simulink model "Par10_3_3S"  (R2018a)
settings: Solver=ode3  StartTime=0.0  StopTime=10.0  FixedStep=0.001  RelTol=1e-3
settings Model: Creator=wangluo  LastModifiedBy=wangluo

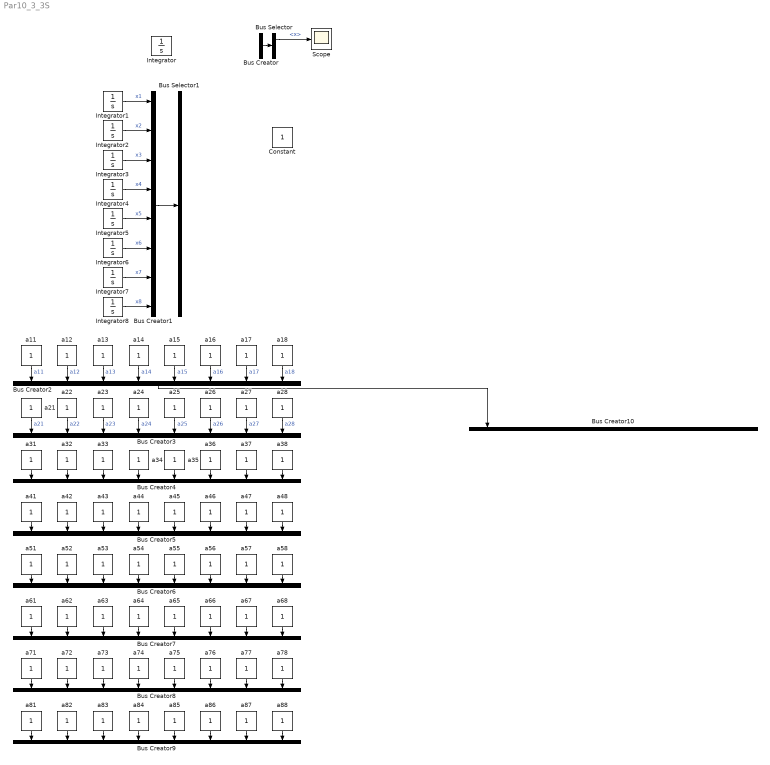
== system Par10_3_3S ==
  Bus Creator : BusCreator  Inputs=2
  Bus Creator{1..10} (10 alike) : BusCreator  Inputs=8
  Bus Selector : BusSelector  OutputSignals=x,signal2
  Bus Selector1 : BusSelector  OutputSignals=x1,x2,x3,x4,x5,x6,x7,x8
  Constant : Constant
  Integrator : Integrator  InitialCondition=[10, 4, 8, 2, 9, 3, 5, 7]
  Integrator{1..8} (8 alike) : Integrator  InitialCondition=[1, 2]
  Scope : Scope
  a{11..18,21..28,31..38,41..48,51..58,61..68,71..78,81..88} (64 alike) : Constant
  wires:
  Bus Selector/1 -> Scope/1  "<x>"
  Bus Creator/1 -> Bus Selector/1
  Integrator1/1 -> Bus Creator1/1  "x1"
  Integrator8/1 -> Bus Creator1/8  "x8"
  Integrator7/1 -> Bus Creator1/7  "x7"
  Integrator6/1 -> Bus Creator1/6  "x6"
  Integrator5/1 -> Bus Creator1/5  "x5"
  Integrator4/1 -> Bus Creator1/4  "x4"
  Integrator3/1 -> Bus Creator1/3  "x3"
  Integrator2/1 -> Bus Creator1/2  "x2"
  Bus Creator1/1 -> Bus Selector1/1
  a11/1 -> Bus Creator2/1  "a11"
  a12/1 -> Bus Creator2/2  "a12"
  a13/1 -> Bus Creator2/3  "a13"
  a14/1 -> Bus Creator2/4  "a14"
  a15/1 -> Bus Creator2/5  "a15"
  a16/1 -> Bus Creator2/6  "a16"
  a17/1 -> Bus Creator2/7  "a17"
  a18/1 -> Bus Creator2/8  "a18"
  a22/1 -> Bus Creator3/2  "a22"
  a24/1 -> Bus Creator3/4  "a24"
  a26/1 -> Bus Creator3/6  "a26"
  a28/1 -> Bus Creator3/8  "a28"
  a25/1 -> Bus Creator3/5  "a25"
  a27/1 -> Bus Creator3/7  "a27"
  a23/1 -> Bus Creator3/3  "a23"
  a21/1 -> Bus Creator3/1  "a21"
  a38/1 -> Bus Creator4/8
  a33/1 -> Bus Creator4/3
  a34/1 -> Bus Creator4/4
  a35/1 -> Bus Creator4/5
  a32/1 -> Bus Creator4/2
  a36/1 -> Bus Creator4/6
  a37/1 -> Bus Creator4/7
  a31/1 -> Bus Creator4/1
  a42/1 -> Bus Creator5/2
  a44/1 -> Bus Creator5/4
  a46/1 -> Bus Creator5/6
  a48/1 -> Bus Creator5/8
  a45/1 -> Bus Creator5/5
  a47/1 -> Bus Creator5/7
  a43/1 -> Bus Creator5/3
  a41/1 -> Bus Creator5/1
  a52/1 -> Bus Creator6/2
  a55/1 -> Bus Creator6/5
  a56/1 -> Bus Creator6/6
  a53/1 -> Bus Creator6/3
  a54/1 -> Bus Creator6/4
  a57/1 -> Bus Creator6/7
  a58/1 -> Bus Creator6/8
  a51/1 -> Bus Creator6/1
  a62/1 -> Bus Creator7/2
  a65/1 -> Bus Creator7/5
  a63/1 -> Bus Creator7/3
  a66/1 -> Bus Creator7/6
  a64/1 -> Bus Creator7/4
  a61/1 -> Bus Creator7/1
  a67/1 -> Bus Creator7/7
  a68/1 -> Bus Creator7/8
  a72/1 -> Bus Creator8/2
  a75/1 -> Bus Creator8/5
  a76/1 -> Bus Creator8/6
  a74/1 -> Bus Creator8/4
  a73/1 -> Bus Creator8/3
  a71/1 -> Bus Creator8/1
  a77/1 -> Bus Creator8/7
  a78/1 -> Bus Creator8/8
  a87/1 -> Bus Creator9/7
  a88/1 -> Bus Creator9/8
  a86/1 -> Bus Creator9/6
  a81/1 -> Bus Creator9/1
  a83/1 -> Bus Creator9/3
  a82/1 -> Bus Creator9/2
  a85/1 -> Bus Creator9/5
  a84/1 -> Bus Creator9/4
  Bus Creator2/1 -> Bus Creator10/1
